simulink model "model_simMech_4DoF"  (Simulink 9.0)
settings: Solver=ode23  StartTime=0.0  StopTime=trajectory.time(end)  RelTol=1e-3  EnableMultiTasking=on
values from neighbouring files (symbols this model uses):
  kinPar = varargin{4}    [forwardDynamicModel.m]    (also in forwardKinematics.m = varargin{2}; inverseDynamicModel.m = varargin{3}; inverseKinematics.m = varargin{2}; inverseKinematics_2.m = varargin{2})
  N = size(DHpar,1)    [forwardDynamicModel.m]    (also in forwardKinematics.m; inverseDynamicModel.m; kinJacobian.m = size(DHparam,1))
  Pvect = [x;y;z]    [interpolaceDat_vcetneOrientace.m]
  s = [s(1:end-1),s_T(i) + v_T(i)*time_int + 1/2*a_T(i)*time_int.^2 + 1/6*jerk(i)*time_int.^3]    [BAVS_genTrajectories.m]    (also in PVA.m = abs(s))
  sol = varargin{3}    [inverseKinematics.m]    (also in inverseKinematics_2.m)
undefined symbols (not defined in the file or in its folder): forwardKinematics, inverseKinematics, Links, trajectory
libraries: serialManipulator_lib x13, mblibv1 x6
settings Model: Creator=MartinSvejda  LastModifiedBy=MartinSvejda
settings DataIOCC: LimitDataPoints=on  SignalLoggingSaveFormat=ModelDataLogs
settings OptimizationCC: InitFltsAndDblsToZero=on
settings DebuggingCC: SaveWithParameterizedLinksMsg=none  SignalResolutionControl=TryResolveAllWithWarning  SolverPrmCheckMsg=warning  MultiTaskDSMMsg=warning  MultiTaskCondExecSysMsg=none  FcnCallInpInsideContextMsg=warning  StrictBusMsg=Warning
settings GRTTargetCC: TargetFcnLib=ansi_tfl_tmw.mat  CombineOutputUpdateFcns=off  GRTInterface=on
settings SimMechanicsCC: VisDuringSimulation=on

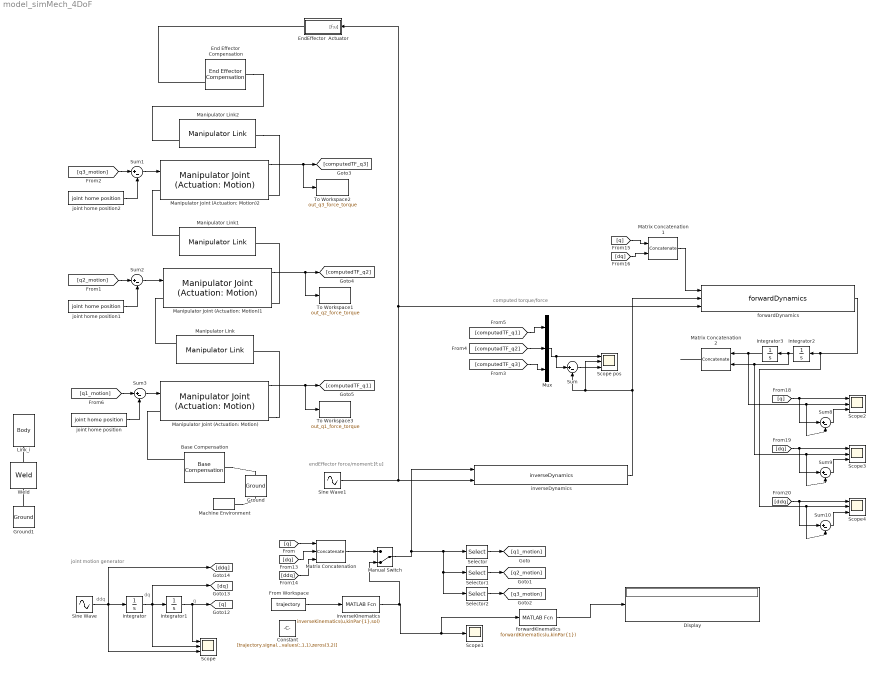
== system model_simMech_4DoF ==
  note: computed torque/force
  note: ddq
  note: dq
  note: q
  note: joint motion generator
  note: endEffector force/moment:[f;u]
  Base Compensation : serialManipulator_lib/Base Compensation  j=1
  Constant : Constant  Value=[trajectory.signals.values(:,1,1),zeros(3,2)]  VectorParams1D=off
  Display : Display
  End Effector Compensation : serialManipulator_lib/End Effector Compensation  j=1
  EndEffector  Actuator : Subsystem
  From Workspace : FromWorkspace  VariableName=trajectory  SampleTime=0  OutputAfterFinalValue=Holding final value
  Ground : mblibv1/Bodies/Ground  UpdateFromCAD=off  LeftPortType=env  RightPortType=workingframe  PhysicalDomain=Mechanical  DialogClass=GroundBlock  CoordPosition=[0;0;0]  CoordPositionUnits=m  StateVectorMgrId=1  MachineId=[3 0]  ShowEnvPort=on  ParameterChecksum=[2407450960, 4092924403, 2530548671, 2904803148]  TopologyChecksum=[1029131939, 1482254733, 934292661, 440378579]
      settings: SourceProductName=Simscape Multibody  SourceProductBaseCode=MS
  Ground1 : mblibv1/Bodies/Ground  UpdateFromCAD=off  LeftPortType=env  RightPortType=workingframe  PhysicalDomain=Mechanical  DialogClass=GroundBlock  CoordPosition=Pvect(:,1)  CoordPositionUnits=m  StateVectorMgrId=2  MachineId=[3 1]  ShowEnvPort=on  ParameterChecksum=[698198439, 3975671620, 1583309806, 644232109]  TopologyChecksum=[1305934639, 3646322005, 772112288, 1061853212]
      settings: SourceProductName=Simscape Multibody  SourceProductBaseCode=MS
  Integrator{,1..3} (4 alike) : Integrator
  Link_i : mblibv1/Bodies/Body  LConnTagsString=CS1  UpdateFromCAD=off  DialogClass=MechanicalBodyBlock  Mass=1e-10  MassUnits=kg  InertiaUnits=kg*m^2  Inertia=1e-10*eye(3)  Shape=Cylinder  ShapeDims=[1 1]  ShapeUnits=m  ShapeUse=false  Density=1  DensityUnits=kg/m^3  DensityUse=false  GraphicsMode=MACHINE_DEFAULT  BodyColorSelMode=MACHINE_DEFAULT  BodyColor=[1 0 0]  AttachedToCS=CG  CG=Left$CG$[0;0;0]$WORLD$WORLD$m$[0;0;0]$Euler X-Y-X$deg$WORLD$false$none  WorkingFrames=Left$CS1$Pvect(:,1)$WORLD$WORLD$m$[0;0;0]$Euler X-Y-X$deg$WORLD$true$none#Right$CS2$Pvect(:,2)$WORLD$WORLD$m$[0;0;0]$Euler X-Y-X$deg$WORLD$false$none#Right$CS3$Pvect(:,3)$WORLD$WORLD$m$[0;0;0]$Euler X-Y-X$deg$WORLD$false$none#Right$CS4$Pvect(:,4)$WORLD$WORLD$m$[0;0;0]$Euler X-Y-X$deg$WORLD$false$none  CGPos=[0;0;0]  CGRot=[0;0;0]  CS0Pos=[]  CS0Rot=[]  CS1Pos=Pvect(:,1)  CS1Rot=[0;0;0]  CS2Pos=Pvect(:,2)  CS2Rot=[0;0;0]  CS3Pos=Pvect(:,3)  CS3Rot=[0;0;0]  CS4Pos=Pvect(:,4)  CS4Rot=[0;0;0]  CS5Pos=[]  CS5Rot=[]  CS6Pos=[]  CS6Rot=[]  CS7Pos=[]  CS7Rot=[]  CS8Pos=[]  CS8Rot=[]  CS9Pos=[]  CS9Rot=[]  CS10Pos=[]  CS10Rot=[]  CS11Pos=[]  CS11Rot=[]  CS12Pos=[]  CS12Rot=[]  CS13Pos=[]  CS13Rot=[]  CS14Pos=[]  CS14Rot=[]  CS15Pos=[]  CS15Rot=[]  CS16Pos=[]  CS16Rot=[]  CS17Pos=[]  CS17Rot=[]  CS18Pos=[]  CS18Rot=[]  CS19Pos=[]  CS19Rot=[]  CS20Pos=[]  CS20Rot=[]
      settings: SourceProductName=Simscape Multibody  SourceProductBaseCode=MS
  Machine Environment : mblibv1/Bodies/Machine Environment  Tag=Factory ground  PortType=env  PhysicalDomain=Mechanical  DialogTemplateClass=MECH.MachineEnvironment  SyncWhenCopied=off  Gravity=Links{1}{1}.gravityVector  GravityUnits=m/s^2  GravityAsSignal=off  Dimensionality=Auto-detect  AnalysisType=Inverse dynamics  LinearAssemblyTolerance=1e-3  LinearAssemblyToleranceUnits=m  AngularAssemblyTolerance=1e-3  AngularAssemblyToleranceUnits=rad  ConstraintSolverType=Stabilizing  ConstraintRelTolerance=1e-4  ConstraintAbsTolerance=1e-4  UseRobustSingularityHandling=off  RedundancyAnalysisToleranceType=Automatically select tolerance  RedundancyAnalysisTolerance=1e-14  StatePerturbationType=Fixed  PerturbationSize=1e-5  VisualizeMachine=on  BodyVisualizationType=Use model default body geometries  BodyColorSelMode=Use model default  DefaultBodyColor=[1 0 0]
      settings: SourceProductName=Simscape Multibody  SourceProductBaseCode=MS
  Manipulator Joint (Actuation: Motion) : serialManipulator_lib/Manipulator Joint (Actuation: Motion)  j=1  i=1
  Manipulator Joint (Actuation: Motion)1 : serialManipulator_lib/Manipulator Joint (Actuation: Motion)  j=1  i=2
  Manipulator Joint (Actuation: Motion)2 : serialManipulator_lib/Manipulator Joint (Actuation: Motion)  j=1  i=3
  Manipulator Link : serialManipulator_lib/Manipulator Link  j=1  i=1
  Manipulator Link1 : serialManipulator_lib/Manipulator Link  j=1  i=2
  Manipulator Link2 : serialManipulator_lib/Manipulator Link  j=1  i=3
  Manual Switch : ManualSwitch  CurrentSetting=0
  Matrix Concatenation : Concatenate  NumInputs=3  Mode=Multidimensional array  ConcatenateDimension=2
  Matrix Concatenation1 : Concatenate  Mode=Multidimensional array  ConcatenateDimension=2
  Matrix Concatenation2 : Concatenate  Mode=Multidimensional array  ConcatenateDimension=2
  Mux : Mux  Inputs=3
  Scope{,2..4} (4 alike) : Scope  NumInputPorts=3
  "Scope pos " : Scope  NumInputPorts=3
  Scope1 : Scope
  Selector : Selector  NumberOfDimensions=2  InputPortWidth=6  IndexOptions=Index vector (dialog),Index vector (dialog)  Indices=1,1:3  OutputSizes=1
  Selector1 : Selector  NumberOfDimensions=2  InputPortWidth=6  IndexOptions=Index vector (dialog),Index vector (dialog)  Indices=2,1:3  OutputSizes=1
  Selector2 : Selector  NumberOfDimensions=2  InputPortWidth=6  IndexOptions=Index vector (dialog),Index vector (dialog)  Indices=3,1:3  OutputSizes=1
  Sine Wave : Sin  Amplitude=[0.6;0.5;0.2]  Bias=[0;0;0]  Frequency=[1;1.2;1.5]  Phase=[0;0.3;0.5]  SampleTime=0  VectorParams1D=off
  Sine Wave1 : Sin  Amplitude=[2;-1;0.8;1;-0.6;-0.8]*0  Bias=[0;0;0;0;0;0]  Frequency=[1;1.2;1;2;0.2;0.1]  Phase=[0;0.3;2;1;2;3]  SampleTime=0  VectorParams1D=off
  Sum{,1..3,8..10} (7 alike) : Sum  Inputs=|+-
  To Workspace1 : ToWorkspace  VariableName=out_q2_force_torque  SaveFormat=Structure With Time  SampleTime=-1
  To Workspace2 : ToWorkspace  VariableName=out_q3_force_torque  SaveFormat=Structure With Time  SampleTime=-1
  To Workspace3 : ToWorkspace  VariableName=out_q1_force_torque  SaveFormat=Structure With Time  SampleTime=-1
  Weld : mblibv1/Joints/Weld  LConnTagsString=__newl0  RConnTagsString=__newr0  UpdateFromCAD=off  NumSAPorts=0  CutJoint=off  MarkAsCut=off  Primitives=weld  PrimitiveProps=W$INERTIAL$[0 0 0]$weld  DialogClass=JointBlock  WAxis=[0 0 0]
      settings: SourceProductName=Simscape Multibody  SourceProductBaseCode=MS
  forwardDynamics : serialManipulator_lib/forwardDynamics
  forwardKinematics : MATLABFcn  MATLABFcn=forwardKinematics(u,kinPar{1})  Output1D=off
  inverseDynamics : serialManipulator_lib/inverseDynamics
  inverseKinematics : MATLABFcn  MATLABFcn=inverseKinematics(u,kinPar{1},sol)  Output1D=off
  joint home position : serialManipulator_lib/joint home position  j=1  i=1
  joint home position1 : serialManipulator_lib/joint home position  j=1  i=2
  joint home position2 : serialManipulator_lib/joint home position  j=1  i=3
  wires:
  Selector/1 -> [q1_motion]
  Selector1/1 -> [q2_motion]
  Matrix Concatenation/1 -> Manual Switch/1
  inverseDynamics/1 -> Sum/2, "Scope pos "/2, forwardDynamics/2
  [q3_motion] -> Sum1/1
  joint home position2/1 -> Sum1/2
  Selector2/1 -> [q3_motion]
  Sum/1 -> "Scope pos "/3
  Sine Wave1/1 -> EndEffector  Actuator/1("[f;u]"), forwardDynamics/3, inverseDynamics/2
  Mux/1 -> Sum/1, "Scope pos "/1
  [computedTF_q3] -> Mux/3
  [computedTF_q2] -> Mux/2
  [computedTF_q1] -> Mux/1
  Manipulator Joint (Actuation: Motion)2/1 -> [computedTF_q3], To Workspace2/1
  Sum1/1 -> Manipulator Joint (Actuation: Motion)2/1
  [q2_motion] -> Sum2/1
  joint home position1/1 -> Sum2/2
  Sum2/1 -> Manipulator Joint (Actuation: Motion)1/1
  [q1_motion] -> Sum3/1
  joint home position/1 -> Sum3/2
  Sum3/1 -> Manipulator Joint (Actuation: Motion)/1
  Manipulator Joint (Actuation: Motion)1/1 -> [computedTF_q2], To Workspace1/1
  Manipulator Joint (Actuation: Motion)/1 -> [computedTF_q1], To Workspace3/1
  Sine Wave/1 -> Integrator/1, Scope/3, [ddq]
  Integrator/1 -> Integrator1/1, Scope/2, [dq]
  Integrator1/1 -> Scope/1, [q]
  [q] -> Matrix Concatenation/1
  [dq] -> Matrix Concatenation/2
  [ddq] -> Matrix Concatenation/3
  forwardDynamics/1 -> Integrator2/1, Scope4/2, Sum10/2
  Integrator2/1 -> Integrator3/1, Matrix Concatenation2/2, Scope3/2, Sum9/2
  Integrator3/1 -> Matrix Concatenation2/1, Sum8/2, Scope2/2
  Sum8/1 -> Scope2/3
  [q] -> Sum8/1, Scope2/1
  Sum9/1 -> Scope3/3
  [dq] -> Scope3/1, Sum9/1
  Sum10/1 -> Scope4/3
  [ddq] -> Scope4/1, Sum10/1
  [q] -> Matrix Concatenation1/1
  [dq] -> Matrix Concatenation1/2
  Matrix Concatenation1/1 -> forwardDynamics/1
  Matrix Concatenation2/1 -> ?
  Manual Switch/1 -> Selector/1, Selector1/1, Selector2/1, inverseDynamics/1
  inverseKinematics/1 -> Manual Switch/2, forwardKinematics/1, Scope1/1
  forwardKinematics/1 -> Display/1
  From Workspace/1 -> inverseKinematics/1
  connections:
  Machine Environment/RConn1 -- Ground/LConn1
  Manipulator Link/RConn1 -- Manipulator Joint (Actuation: Motion)1/LConn1
  End Effector Compensation/RConn2 -- EndEffector  Actuator/RConn1
  Manipulator Joint (Actuation: Motion)/RConn1 -- Manipulator Link/LConn1
  Manipulator Joint (Actuation: Motion)1/RConn1 -- Manipulator Link1/LConn1
  Manipulator Link1/RConn1 -- Manipulator Joint (Actuation: Motion)2/LConn1
  Manipulator Link2/LConn1 -- Manipulator Joint (Actuation: Motion)2/RConn1
  Base Compensation/RConn1 -- Manipulator Joint (Actuation: Motion)/LConn1
  Base Compensation/LConn1 -- Ground/RConn1
  End Effector Compensation/LConn1 -- Manipulator Link2/RConn2
  Weld/RConn1 -- Link_i/LConn1
  Ground1/RConn1 -- Weld/LConn1

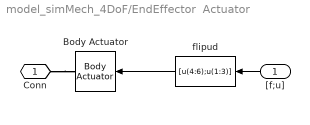
== system model_simMech_4DoF/EndEffector  Actuator ==
  "[f;u]" : Inport
  Body Actuator : mblibv1/Sensors &  Actuators/Body Actuator  UpdateFromCAD=off  PhysicalDomain=Mechanical  PortType=blob  ActuationStyle=Force  AngleUnits=deg  ArcVelocityUnits=deg/s  ArcAccelerationUnits=deg/s^2  CoordPositionUnits=m  VelocityUnits=m/s  AccelerationUnits=m/s^2  ForceUnits=N  TorqueUnits=N-m  ActiveIO=on  Width=6  DialogClass=MechanicalActuatorBlock  ReferenceFrame=Absolute (World)  Angle=off  CoordPosition=on  Force=on  Torque=on
      settings: SourceProductName=Simscape Multibody  SourceProductBaseCode=MS
  flipud : MATLABFcn  MATLABFcn=[u(4:6);u(1:3)]  Output1D=off
  Conn : PMIOPort  Port=1  Side=Right
  wires:
  flipud/1 -> Body Actuator/1
  "[f;u]"/1 -> flipud/1
  connections:
  Conn/RConn1 -- Body Actuator/RConn1
